simulink model "ManufacturingFacility_Alt"  (R2018b)
settings: Solver=VariableStepAuto  StartTime=0.0  StopTime=4000  RelTol=1e-3
undefined symbols (not defined in the file): m, n
settings Model: Creator=Ryan  LastModifiedBy=Ryan

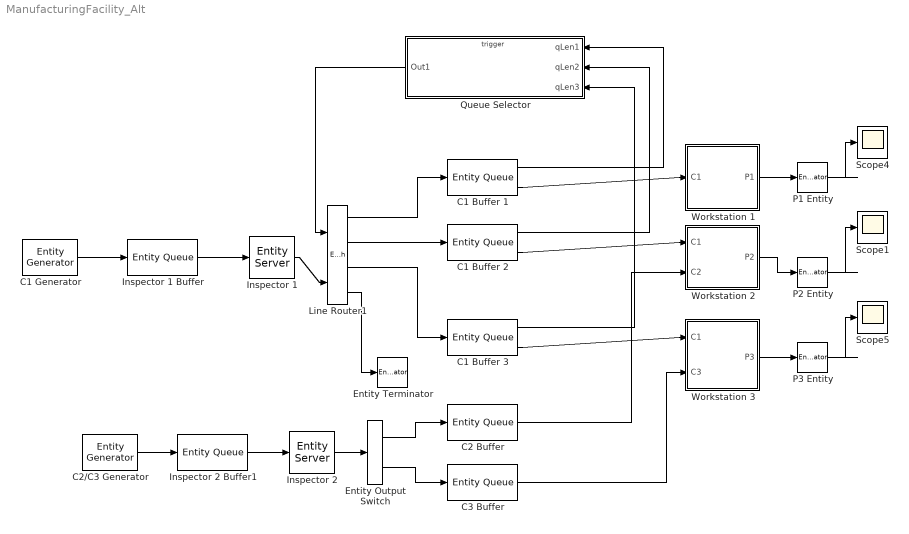
== system ManufacturingFacility_Alt ==
  C1 Buffer 1 : EntityQueue  InputPortMessageModes=m  OutputPortMessageModes=n,m  Capacity=2  NumberEntitiesInBlock=on
      settings: OutputPortMap=o1,o5
  C1 Buffer 2 : EntityQueue  InputPortMessageModes=m  OutputPortMessageModes=n,m  Capacity=2  NumberEntitiesInBlock=on
      settings: OutputPortMap=o1,o5
  C1 Buffer 3 : EntityQueue  InputPortMessageModes=m  OutputPortMessageModes=n,m  Capacity=2  NumberEntitiesInBlock=on
      settings: OutputPortMap=o1,o5
  C1 Generator : EntityGenerator  OutputPortMessageModes=m  Period=0  AttributeName=entityType|outputPort  AttributeInitialValue=1|1  EntityType=Structured  EntityTypeName=Entity
  C2 Buffer : EntityQueue  InputPortMessageModes=m  OutputPortMessageModes=m  Capacity=2
      settings: OutputPortMap=o5
  C2/C3 Generator : EntityGenerator  OutputPortMessageModes=m  Period=0  GenerateAction=|  AttributeName=entityType|outputPort  AttributeInitialValue=1|1  EntityType=Structured  EntityTypeName=Entity
      | % Generate a random entity type corresponding
      | % To the component type
      | entity.entityType = randi([2, 3])
      | 
      | % Define the output port
      | switch entity.entityType
      |     case 2
      |         entity.outputPort = 1
      |     case 3
      |         entity.outputPort = 2
      |     otherwise
      |         error('Invalid entity type')
      | end
  C3 Buffer : EntityQueue  InputPortMessageModes=m  OutputPortMessageModes=m  Capacity=2
      settings: OutputPortMap=o5
  Entity Output Switch : EntityOutputSwitch  InputPortMessageModes=m  OutputPortMessageModes=m,m  SwitchingCriterion=From attribute  SwitchAttributeName=outputPort
  Entity Terminator : EntityTerminator  InputPortMessageModes=m
  Inspector 1 : EntityServer  InputPortMessageModes=m  OutputPortMessageModes=m  Capacity=1  ServiceTimeSource=MATLAB action  ServiceTimeAction=dt = wblrnd(10.725, 1.096);  EntryAction=|
      | % Entity will select the shortest queue
      | pickRandomQueue();
  Inspector 1 Buffer : EntityQueue  InputPortMessageModes=m  OutputPortMessageModes=m
      settings: OutputPortMap=o5
  "Inspector 2 " : EntityServer  InputPortMessageModes=m  OutputPortMessageModes=m  Capacity=1  ServiceTimeSource=MATLAB action  ServiceTimeAction=|
      | % Depending on the type of entity
      | % Generate the appropriate service time
      | switch entity.entityType
      |     case 2
      |         dt = wblrnd(16.0876, 1.09601);
      |     case 3
      |         dt = exprnd(20.6328);
      |     otherwise
      |         dt = -1
      | end
  Inspector 2 Buffer1 : EntityQueue  InputPortMessageModes=m  OutputPortMessageModes=m
      settings: OutputPortMap=o5
  Line Router1 : EntityOutputSwitch  InputPortMessageModes=m,m  OutputPortMessageModes=m,m,m,m  NumberOutputPorts=4  SwitchingCriterion=From control port  SwitchAttributeName=QueuePath
      settings: InputPortMap=u0,u1  OutputPortMap=o0,o1,o2,o3
  P1 Entity : EntityTerminator  InputPortMessageModes=m  NumberEntitiesArrived=on
      settings: OutputPortMap=o0
  P2 Entity : EntityTerminator  InputPortMessageModes=m  NumberEntitiesArrived=on
      settings: OutputPortMap=o0
  P3 Entity : EntityTerminator  InputPortMessageModes=m  NumberEntitiesArrived=on
      settings: OutputPortMap=o0
  Queue Selector : Subsystem  TreatAsAtomicUnit=on
  Scope1 : Scope
  Scope4 : Scope
  Scope5 : Scope
  "Workstation 1 " : Subsystem
  Workstation 2 : Subsystem
  Workstation 3 : Subsystem
  wires:
  "Inspector 2 "/1 -> Entity Output Switch/1
  Entity Output Switch/1 -> C2 Buffer/1
  C1 Buffer 2/2 -> Workstation 2/1(C1)
  P2 Entity/1 -> Scope1/1
  P1 Entity/1 -> Scope4/1
  Inspector 2 Buffer1/1 -> "Inspector 2 "/1
  Line Router1/1 -> C1 Buffer 1/1
  "Workstation 1 "/1(P1) -> P1 Entity/1
  C3 Buffer/1 -> Workstation 3/2(C3)
  Entity Output Switch/2 -> C3 Buffer/1
  C1 Buffer 1/1 -> Queue Selector/1(qLen1)
  C1 Buffer 1/2 -> "Workstation 1 "/1(C1)
  Line Router1/2 -> C1 Buffer 2/1
  Inspector 1/1 -> Line Router1/2
  Queue Selector/1(Out1) -> Line Router1/1
  Workstation 3/1(P3) -> P3 Entity/1
  Inspector 1 Buffer/1 -> Inspector 1/1
  C1 Generator/1 -> Inspector 1 Buffer/1
  C1 Buffer 3/1 -> Queue Selector/3(qLen3)
  C1 Buffer 3/2 -> Workstation 3/1(C1)
  C1 Buffer 2/1 -> Queue Selector/2(qLen2)
  Workstation 2/1(P2) -> P2 Entity/1
  C2 Buffer/1 -> Workstation 2/2(C2)
  C2/C3 Generator/1 -> Inspector 2 Buffer1/1
  P3 Entity/1 -> Scope5/1
  Line Router1/4 -> Entity Terminator/1
  Line Router1/3 -> C1 Buffer 3/1

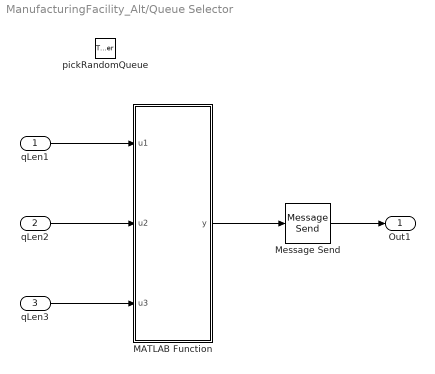
== system ManufacturingFacility_Alt/Queue Selector ==
  qLen1 : Inport
  qLen2 : Inport  Port=2
  qLen3 : Inport  Port=3
  pickRandomQueue : TriggerPort  TriggerType=function-call  IsSimulinkFunction=on  FunctionName=pickRandomQueue  FunctionVisibility=scoped  VariantControl=Variant
  MATLAB Function : MATLAB Function  TreatAsAtomicUnit=on
  Message Send : MessageSend  OutputPortMessageModes=m
      settings: InputPortMap=u1
  Out1 : Outport
  wires:
  qLen1/1 -> MATLAB Function/1(u1)
  qLen2/1 -> MATLAB Function/2(u2)
  qLen3/1 -> MATLAB Function/3(u3)
  MATLAB Function/1(y) -> Message Send/1
  Message Send/1 -> Out1/1

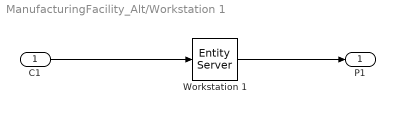
== system ManufacturingFacility_Alt/Workstation 1  ==
  C1 : Inport
  Workstation 1 : EntityServer  InputPortMessageModes=m  OutputPortMessageModes=m  Capacity=1  ServiceTimeSource=MATLAB action  ServiceTimeValue=20  ServiceTimeAction=dt = exprnd(4.60442);
  P1 : Outport
  wires:
  Workstation 1/1 -> P1/1
  C1/1 -> Workstation 1/1

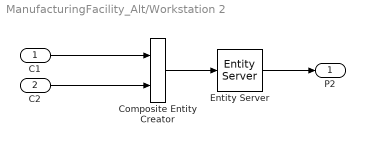
== system ManufacturingFacility_Alt/Workstation 2 ==
  C1 : Inport
  C2 : Inport  Port=2
  Composite Entity Creator : CompositeEntityCreator  InputPortMessageModes=m,m  OutputPortMessageModes=m  EntityTypeName=Combined
      settings: InputPortMap=u0,u1
  Entity Server : EntityServer  InputPortMessageModes=m  OutputPortMessageModes=m  Capacity=1  ServiceTimeSource=MATLAB action  ServiceTimeValue=20  ServiceTimeAction=dt = wblrnd(10.6815, 0.922808);
  P2 : Outport
  wires:
  C2/1 -> Composite Entity Creator/2
  Composite Entity Creator/1 -> Entity Server/1
  Entity Server/1 -> P2/1
  C1/1 -> Composite Entity Creator/1

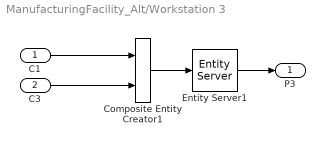
== system ManufacturingFacility_Alt/Workstation 3 ==
  C1 : Inport
  C3 : Inport  Port=2
  Composite Entity Creator1 : CompositeEntityCreator  InputPortMessageModes=m,m  OutputPortMessageModes=m  EntityTypeName=Combined
      settings: InputPortMap=u0,u1
  Entity Server1 : EntityServer  InputPortMessageModes=m  OutputPortMessageModes=m  Capacity=1  ServiceTimeSource=MATLAB action  ServiceTimeValue=20  ServiceTimeAction=dt = exprnd(8.79558);
  P3 : Outport
  wires:
  Entity Server1/1 -> P3/1
  C3/1 -> Composite Entity Creator1/2
  Composite Entity Creator1/1 -> Entity Server1/1
  C1/1 -> Composite Entity Creator1/1

== matlab function ManufacturingFacility_Alt/Queue Selector/MATLAB Function ==
  data: u1 input; y output; u2 input; u3 input
function y = fcn(u1, u2, u3)
y = randi([1,3]);
if and(y == 1, u1 >= 2) || and(y==2, u2 >=2) || and(y==3, u3 >=2)
    y = 4;
end
